simulink model "CORRECTO_REGULADOR"  (R2019b)
settings: Solver=VariableStepAuto  StartTime=0.0  StopTime=50000  RelTol=1e-3
undefined symbols (not defined in the file): n, p1, p2, p3, p6, Vi
libraries: simulink x39
(part 1 of 2)
settings Model: Creator=USUARIO  LastModifiedBy=USUARIO

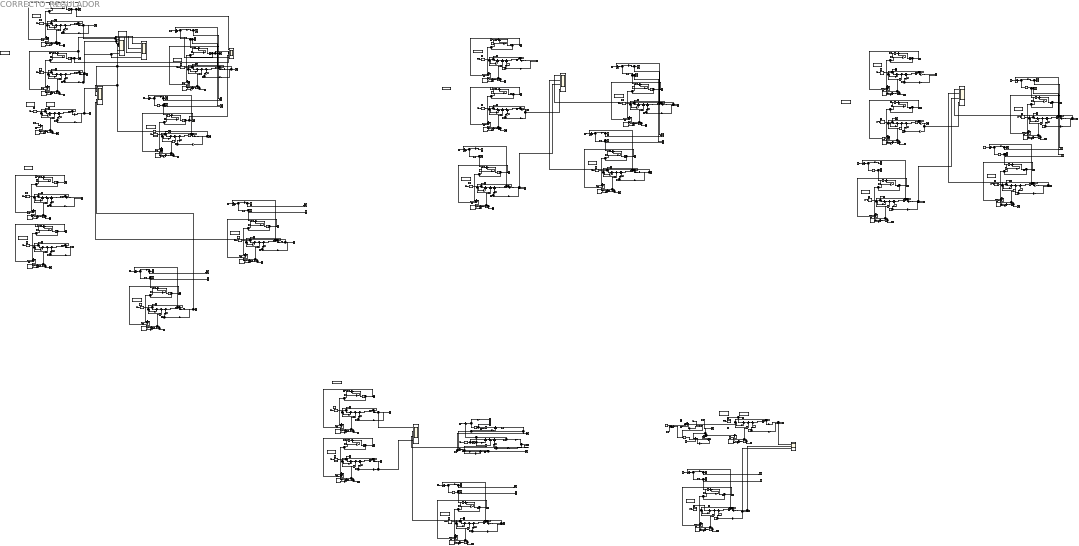
== system CORRECTO_REGULADOR ==
  Clock{,1..25} (26 alike) : Clock
  Constant{1,3,5..7,9,11,15,17,19,21,24,26,28,31,35,37,39,41..43,45..46,48} (24 alike) : Constant  Value=0
  Constant{2,4,8,10,12..14,16,18,20,22..23,25,27,30,32..34,36,38,40,44,47} (23 alike) : Constant  Value=Vi
  Divide{1..23} (23 alike) : Product  Inputs=*/
  Error glucémico{,1,3..4,6,8,12..15,17,19} (12 alike) : Scope
  "Error glucémico   " : Scope
  Error glucémico{2,5,7,9,16,18,20} (7 alike) : Scope  NumInputPorts=2
  Gain{1,6,8,10,15,17,23,26,31,35,37,41,44,52..53,57,63..64,68,73,76,80,83,88,91,95,100,103,105,110,113,118,121,126,129,134,141..142,146,152,155..156,159,164,167,171,173,178,181,185} (50 alike) : Gain  Gain=p1
  Gain{7,16,24,42,45..46,59,74,77..78,81,89,101,104,111,119,127,135,148,153,157,165,172,179,186} (25 alike) : Gain  Gain=p2
  Gain{3,5,9,12,14,18,20,22,25,28,30,33,38,40,43,47,49,51,55,60,62,66,70,72,75,79,82,85,87,90,93,97,99,102,107,109,112,115,117,120,123,125,128,131,133,136,138,140,144,149,151,154,158,161,163,166,169..170,175,177,180,183..184} (63 alike) : Gain  Gain=18
  Gain{2,11,19,27,32,36,48,54,58,65,69,84,92,96,106,114,122,130,137,143,147,160,168,174,182} (25 alike) : Gain  Gain=p3
  Gain{4,13,21,29,34,39,50,56,61,67,71,86,94,98,108,116,124,132,139,145,150,162,176} (23 alike) : Gain  Gain=n
  "Glucosa " : Constant  Value=10
  "Glucosa basal     " : Constant  Value=7
  Glucosa basal{1..14,16..22} (21 alike) : Constant  Value=7
  Glucosa basal23 : Constant  Value=4.5
  Glucosa basal24 : Constant  Value=6
  Glucosa basal25 : Constant  Value=6
  Glucosa basal26 : Constant
  Glucosa basal27 : Constant  Value=0
  Glucosa con regulador : Scope  NumInputPorts=4
  Grafica ingesta D{1..14,16..25} (24 alike) : Scope
  Gráfica de la glucosa : Scope  NumInputPorts=2
  Gráfica de la ingesta : Scope
  Gráfica de la insulina : Scope  NumInputPorts=2
  Gráfica de la insulina activa : Scope
  INSULINA : Scope  NumInputPorts=2
  Ib : Constant  Value=10
  "Ingesta    " : MATLAB Function  TreatAsAtomicUnit=on
  Ingesta 75 g1 : MATLAB Function  TreatAsAtomicUnit=on
  Ingesta 75 g10 : MATLAB Function  TreatAsAtomicUnit=on
  Ingesta 75 g11 : MATLAB Function  TreatAsAtomicUnit=on
  Ingesta 75 g12 : MATLAB Function  TreatAsAtomicUnit=on
  Ingesta 75 g13 : MATLAB Function  TreatAsAtomicUnit=on
  Ingesta 75 g14 : MATLAB Function  TreatAsAtomicUnit=on
  Ingesta 75 g16 : MATLAB Function  TreatAsAtomicUnit=on
  Ingesta 75 g17 : MATLAB Function  TreatAsAtomicUnit=on
  Ingesta 75 g18 : MATLAB Function  TreatAsAtomicUnit=on
  Ingesta 75 g19 : MATLAB Function  TreatAsAtomicUnit=on
  Ingesta 75 g2 : MATLAB Function  TreatAsAtomicUnit=on
  Ingesta 75 g20 : MATLAB Function  TreatAsAtomicUnit=on
  Ingesta 75 g21 : MATLAB Function  TreatAsAtomicUnit=on
  Ingesta 75 g22 : MATLAB Function  TreatAsAtomicUnit=on
  Ingesta 75 g23 : MATLAB Function  TreatAsAtomicUnit=on
  Ingesta 75 g24 : MATLAB Function  TreatAsAtomicUnit=on
  Ingesta 75 g25 : MATLAB Function  TreatAsAtomicUnit=on
  Ingesta 75 g3 : MATLAB Function  TreatAsAtomicUnit=on
  Ingesta 75 g4 : MATLAB Function  TreatAsAtomicUnit=on
  Ingesta 75 g5 : MATLAB Function  TreatAsAtomicUnit=on
  Ingesta 75 g6 : MATLAB Function  TreatAsAtomicUnit=on
  Ingesta 75 g7 : MATLAB Function  TreatAsAtomicUnit=on
  Ingesta 75 g8 : MATLAB Function  TreatAsAtomicUnit=on
  Ingesta 75 g9 : MATLAB Function  TreatAsAtomicUnit=on
  "Insulina basal     " : Constant  Value=10
  Insulina basal{1..14,16..22,24..25} (23 alike) : Constant  Value=10
  Insulina basal23 : Constant  Value=12
  Integrator{1,4,7,9,11,13,16,22,25,28,31,36,39,42..43,46,49,53,56,59,62,64,69} (23 alike) : Integrator  InitialCondition=10
  Integrator{2,5,8,10,14,17,19,23,26,29,32,34,37,40,44,47,50,54,57,60,63,65} (22 alike) : Integrator  InitialCondition=7
  Integrator{3,6,12,18,20..21,27,30,35,41,45,48,51..52,58,61,66,68,71,74} (20 alike) : Integrator
  Integrator{15,24,33,38,55} (5 alike) : Integrator  InitialCondition=-0.000194
  Integrator67 : Integrator  InitialCondition=4.5
  Integrator70 : Integrator  InitialCondition=9.5
  Integrator72 : Integrator  InitialCondition=9.5
  Integrator73 : Integrator  InitialCondition=12
  Model Info1 : simulink/Model-Wide Utilities/Model Info  Frame=on  DisplayStringWithTags=|  HorizontalTextAlignment=Center  LeftAlignmentValue=0.5
      | MODELO MODIFICADO
      | 
      | INGESTA SIN INSULINA
      | 
      | PERSONA DIABETICA tipo 1
  Model Info10 : simulink/Model-Wide Utilities/Model Info  Frame=on  DisplayStringWithTags=|  HorizontalTextAlignment=Center  LeftAlignmentValue=0.5
      | MODELO MODIFICADO
      | 
      | TRAS INGESTA CON INSULINA
      | 
      | PERSONA DIABETICA
  Model Info11 : simulink/Model-Wide Utilities/Model Info  Frame=on  DisplayStringWithTags=|  HorizontalTextAlignment=Center  LeftAlignmentValue=0.5
      | MODELO MODIFICADO
      | 
      | INGESTA SIN INSULINA
      | 
      | PERSONA DIABETICA tipo 1
  Model Info12 : simulink/Model-Wide Utilities/Model Info  Frame=on  DisplayStringWithTags=|  HorizontalTextAlignment=Center  LeftAlignmentValue=0.5
      | MODELO MODIFICADO
      | 
      | INGESTA SIN INSULINA
      | 
      | PERSONA DIABETICA tipo 1
  Model Info13 : simulink/Model-Wide Utilities/Model Info  Frame=on  DisplayStringWithTags=PRUEBA Y ERROR  HorizontalTextAlignment=Center  LeftAlignmentValue=0.5
  Model Info15 : simulink/Model-Wide Utilities/Model Info  Frame=on  DisplayStringWithTags=|  HorizontalTextAlignment=Center  LeftAlignmentValue=0.5
      | MODELO MODIFICADO
      | 
      | INGESTA SIN INSULINA
      | 
      | PERSONA DIABETICA tipo 1
  Model Info16 : simulink/Model-Wide Utilities/Model Info  Frame=on  DisplayStringWithTags=|  HorizontalTextAlignment=Center  LeftAlignmentValue=0.5
      | MODELO MODIFICADO
      | 
      | INGESTA SIN INSULINA
      | 
      | PERSONA DIABETICA tipo 1
  Model Info17 : simulink/Model-Wide Utilities/Model Info  Frame=on  DisplayStringWithTags=|  HorizontalTextAlignment=Center  LeftAlignmentValue=0.5
      | MODELO MODIFICADO
      | 
      | INGESTA SIN INSULINA
      | 
      | PERSONA DIABETICA tipo 1
  Model Info18 : simulink/Model-Wide Utilities/Model Info  Frame=on  DisplayStringWithTags=|  HorizontalTextAlignment=Center  LeftAlignmentValue=0.5
      | MODELO MODIFICADO
      | 
      | INGESTA SIN INSULINA
      | 
      | PERSONA DIABETICA tipo 1
  Model Info19 : simulink/Model-Wide Utilities/Model Info  Frame=on  DisplayStringWithTags=|  HorizontalTextAlignment=Center  LeftAlignmentValue=0.5
      | MODELO MODIFICADO
      | 
      | INGESTA SIN INSULINA
      | 
      | PERSONA DIABETICA tipo 1
  Model Info2 : simulink/Model-Wide Utilities/Model Info  Frame=on  DisplayStringWithTags=|  HorizontalTextAlignment=Center  LeftAlignmentValue=0.5
      | MODELO MODIFICADO
      | 
      | INGESTA SIN INSULINA
      | 
      | PERSONA DIABETICA tipo 1
  Model Info20 : simulink/Model-Wide Utilities/Model Info  Frame=on  DisplayStringWithTags=|  HorizontalTextAlignment=Center  LeftAlignmentValue=0.5
      | MODELO MODIFICADO
      | 
      | INGESTA SIN INSULINA
      | 
      | PERSONA DIABETICA tipo 1
  Model Info21 : simulink/Model-Wide Utilities/Model Info  Frame=on  DisplayStringWithTags=VARIACION TÉRMINO I  HorizontalTextAlignment=Center  LeftAlignmentValue=0.5
  Model Info22 : simulink/Model-Wide Utilities/Model Info  Frame=on  DisplayStringWithTags=|  HorizontalTextAlignment=Center  LeftAlignmentValue=0.5
      | MODELO MODIFICADO
      | 
      | INGESTA SIN INSULINA
      | 
      | PERSONA DIABETICA tipo 1
  Model Info23 : simulink/Model-Wide Utilities/Model Info  Frame=on  DisplayStringWithTags=|  HorizontalTextAlignment=Center  LeftAlignmentValue=0.5
      | Insulina constante 
      | igual a la basal
      | 
      | I(0) = Ib
  Model Info24 : simulink/Model-Wide Utilities/Model Info  Frame=on  DisplayStringWithTags=|  HorizontalTextAlignment=Center  LeftAlignmentValue=0.5
      | MODELO ORIGINAL
      | 
      | 
      | PERSONA NO DIABETICA
      | 
      | CON INSULINA CONSTANTE
  Model Info25 : simulink/Model-Wide Utilities/Model Info  Frame=on  DisplayStringWithTags=|  HorizontalTextAlignment=Center  LeftAlignmentValue=0.5
      | MODELO MODIFICADO
      | 
      | INGESTA SIN INSULINA
      | 
      | PERSONA DIABETICA tipo 1
  Model Info26 : simulink/Model-Wide Utilities/Model Info  Frame=on  DisplayStringWithTags=|  HorizontalTextAlignment=Center  LeftAlignmentValue=0.5
      | Insulina constante 
      | igual a la basal
      | 
      | I(0) = Ib
  Model Info27 : simulink/Model-Wide Utilities/Model Info  Frame=on  DisplayStringWithTags=|  HorizontalTextAlignment=Center  LeftAlignmentValue=0.5
      | MODELO ORIGINAL
      | 
      | 
      | PERSONA NO DIABETICA
      | 
      | CON INSULINA VARIABLE
  Model Info3 : simulink/Model-Wide Utilities/Model Info  Frame=on  DisplayStringWithTags=|  HorizontalTextAlignment=Center  LeftAlignmentValue=0.5
      | MODELO MODIFICADO
      | 
      | INGESTA SIN INSULINA
      | 
      | PERSONA DIABETICA tipo 1
  Model Info4 : simulink/Model-Wide Utilities/Model Info  Frame=on  DisplayStringWithTags=REGULADOR SINTONIZADO  HorizontalTextAlignment=Center  LeftAlignmentValue=0.5
  Model Info5 : simulink/Model-Wide Utilities/Model Info  Frame=on  DisplayStringWithTags=|  HorizontalTextAlignment=Center  LeftAlignmentValue=0.5
      | MODELO MODIFICADO
      | 
      | TRAS INGESTA CON INSULINA
      | 
      | PERSONA DIABETICA
  Model Info6 : simulink/Model-Wide Utilities/Model Info  Frame=on  DisplayStringWithTags=|  HorizontalTextAlignment=Center  LeftAlignmentValue=0.5
      | MODELO MODIFICADO
      | 
      | INGESTA SIN INSULINA
      | 
      | PERSONA DIABETICA tipo 1
  Model Info7 : simulink/Model-Wide Utilities/Model Info  Frame=on  DisplayStringWithTags=|  HorizontalTextAlignment=Center  LeftAlignmentValue=0.5
      | MODELO MODIFICADO
      | 
      | INGESTA SIN INSULINA
      | 
      | PERSONA DIABETICA tipo 1
  Model Info8 : simulink/Model-Wide Utilities/Model Info  Frame=on  DisplayStringWithTags=VARAICION TERMINO P  HorizontalTextAlignment=Center  LeftAlignmentValue=0.5
  Model Info9 : simulink/Model-Wide Utilities/Model Info  Frame=on  DisplayStringWithTags=REGULADOR SINTONIZADO  HorizontalTextAlignment=Center  LeftAlignmentValue=0.5
  PID Controller : simulink/Continuous/PID Controller  Controller=PID  Form=Ideal  TimeDomain=Continuous-time  SampleTime=-1  IntegratorMethod=Forward Euler  FilterMethod=Forward Euler  ControllerParametersSource=internal  P=-0.4  I=0  D=0  UseFilter=on  N=10  TunerSelectOption=Transfer Function Based (PID Tuner App)  InitialConditionSource=internal  InitialConditionForIntegrator=-0.1  InitialConditionForFilter=0  DifferentiatorICPrevScaledInput=0  ExternalReset=none  TrackingMode=off  Kt=1  LimitOutput=off  UpperSaturationLimit=inf  LowerSaturationLimit=-inf  LinearizeAsGain=on  AntiWindupMode=none  Kb=1  POutMin=[]  POutMax=[]  IOutMin=[]  IOutMax=[]  DOutMin=[]  DOutMax=[]  NOutMin=[]  NOutMax=[]  SumOutMin=[]  SumOutMax=[]  SaturationOutMin=[]  SaturationOutMax=[]  PParamMin=[]  PParamMax=[]  IParamMin=[]  IParamMax=[]  DParamMin=[]  DParamMax=[]  NParamMin=[]  NParamMax=[]  KbParamMin=[]  KbParamMax=[]  KtParamMin=[]  KtParamMax=[]  KbOutMin=[]  KbOutMax=[]  KtOutMin=[]  KtOutMax=[]  IntegratorOutMin=[]  IntegratorOutMax=[]  FilterOutMin=[]  FilterOutMax=[]  SumI1OutMin=[]  SumI1OutMax=[]  SumI2OutMin=[]  SumI2OutMax=[]  SumI3OutMin=[]  SumI3OutMax=[]  SumI4OutMin=[]  SumI4OutMax=[]  SumDOutMin=[]  SumDOutMax=[]  DifferentiatorOutMin=[]  DifferentiatorOutMax=[]  FilterDiffOutCoefMin=[]  FilterDiffOutCoefMax=[]  ReciprocalOutMin=[]  ReciprocalOutMax=[]  SumDenOutMin=[]  SumDenOutMax=[]  SumNumOutMin=[]  SumNumOutMax=[]  DivideOutMin=[]  DivideOutMax=[]  IntegratorContinuousStateAttributes=''  IntegratorStateMustResolveToSignalObject=off  IntegratorRTWStateStorageClass=Auto  FilterContinuousStateAttributes=''  FilterStateMustResolveToSignalObject=off  FilterRTWStateStorageClass=Auto  ParallelPVariant=Passthrough  IdealPVariant=InternalParameters  IVariant=InternalParameters  DVariant=InternalParameters  IntegratorVariant=Continuous  SatVariant=Disabled  AWVariant=Passthrough  PCopyVariant=Disabled  TRVariant=Disabled  FdbkBlocksVariant=Forward  IdealPFdbkVariant=Disabled  SatFdbkVariant=Disabled  DerivativeFilterVariant=ContFilter  NVariant=InternalParameters  NCopyVariant=Disabled  FilterICVariant=InternalICsFilter  IntegratorICVariant=InternalICs  ExternalResetVariant=Disabled  TRSumVariant=Passthrough  SumFdbkVariant=Disabled  SumVariant=Sum_PID
  PID Controller1 : simulink/Continuous/PID Controller  Controller=PID  Form=Ideal  TimeDomain=Continuous-time  SampleTime=-1  IntegratorMethod=Forward Euler  FilterMethod=Forward Euler  ControllerParametersSource=internal  P=-0.4  I=0.00006  D=0  UseFilter=on  N=100  TunerSelectOption=Transfer Function Based (PID Tuner App)  InitialConditionSource=internal  InitialConditionForIntegrator=-0.1  InitialConditionForFilter=0  DifferentiatorICPrevScaledInput=0  ExternalReset=none  TrackingMode=off  Kt=1  LimitOutput=off  UpperSaturationLimit=inf  LowerSaturationLimit=-inf  LinearizeAsGain=on  AntiWindupMode=none  Kb=1  POutMin=[]  POutMax=[]  IOutMin=[]  IOutMax=[]  DOutMin=[]  DOutMax=[]  NOutMin=[]  NOutMax=[]  SumOutMin=[]  SumOutMax=[]  SaturationOutMin=[]  SaturationOutMax=[]  PParamMin=[]  PParamMax=[]  IParamMin=[]  IParamMax=[]  DParamMin=[]  DParamMax=[]  NParamMin=[]  NParamMax=[]  KbParamMin=[]  KbParamMax=[]  KtParamMin=[]  KtParamMax=[]  KbOutMin=[]  KbOutMax=[]  KtOutMin=[]  KtOutMax=[]  IntegratorOutMin=[]  IntegratorOutMax=[]  FilterOutMin=[]  FilterOutMax=[]  SumI1OutMin=[]  SumI1OutMax=[]  SumI2OutMin=[]  SumI2OutMax=[]  SumI3OutMin=[]  SumI3OutMax=[]  SumI4OutMin=[]  SumI4OutMax=[]  SumDOutMin=[]  SumDOutMax=[]  DifferentiatorOutMin=[]  DifferentiatorOutMax=[]  FilterDiffOutCoefMin=[]  FilterDiffOutCoefMax=[]  ReciprocalOutMin=[]  ReciprocalOutMax=[]  SumDenOutMin=[]  SumDenOutMax=[]  SumNumOutMin=[]  SumNumOutMax=[]  DivideOutMin=[]  DivideOutMax=[]  IntegratorContinuousStateAttributes=''  IntegratorStateMustResolveToSignalObject=off  IntegratorRTWStateStorageClass=Auto  FilterContinuousStateAttributes=''  FilterStateMustResolveToSignalObject=off  FilterRTWStateStorageClass=Auto  ParallelPVariant=Passthrough  IdealPVariant=InternalParameters  IVariant=InternalParameters  DVariant=InternalParameters  IntegratorVariant=Continuous  SatVariant=Disabled  AWVariant=Passthrough  PCopyVariant=Disabled  TRVariant=Disabled  FdbkBlocksVariant=Forward  IdealPFdbkVariant=Disabled  SatFdbkVariant=Disabled  DerivativeFilterVariant=ContFilter  NVariant=InternalParameters  NCopyVariant=Disabled  FilterICVariant=InternalICsFilter  IntegratorICVariant=InternalICs  ExternalResetVariant=Disabled  TRSumVariant=Passthrough  SumFdbkVariant=Disabled  SumVariant=Sum_PID
  PID Controller10 : simulink/Continuous/PID Controller  Controller=PID  Form=Ideal  TimeDomain=Continuous-time  SampleTime=-1  IntegratorMethod=Forward Euler  FilterMethod=Forward Euler  ControllerParametersSource=internal  P=-0.4  I=0.00001  D=0  UseFilter=on  N=100  TunerSelectOption=Transfer Function Based (PID Tuner App)  InitialConditionSource=internal  InitialConditionForIntegrator=-0.1  InitialConditionForFilter=0  DifferentiatorICPrevScaledInput=0  ExternalReset=none  TrackingMode=off  Kt=1  LimitOutput=off  UpperSaturationLimit=inf  LowerSaturationLimit=-inf  LinearizeAsGain=on  AntiWindupMode=none  Kb=1  POutMin=[]  POutMax=[]  IOutMin=[]  IOutMax=[]  DOutMin=[]  DOutMax=[]  NOutMin=[]  NOutMax=[]  SumOutMin=[]  SumOutMax=[]  SaturationOutMin=[]  SaturationOutMax=[]  PParamMin=[]  PParamMax=[]  IParamMin=[]  IParamMax=[]  DParamMin=[]  DParamMax=[]  NParamMin=[]  NParamMax=[]  KbParamMin=[]  KbParamMax=[]  KtParamMin=[]  KtParamMax=[]  KbOutMin=[]  KbOutMax=[]  KtOutMin=[]  KtOutMax=[]  IntegratorOutMin=[]  IntegratorOutMax=[]  FilterOutMin=[]  FilterOutMax=[]  SumI1OutMin=[]  SumI1OutMax=[]  SumI2OutMin=[]  SumI2OutMax=[]  SumI3OutMin=[]  SumI3OutMax=[]  SumI4OutMin=[]  SumI4OutMax=[]  SumDOutMin=[]  SumDOutMax=[]  DifferentiatorOutMin=[]  DifferentiatorOutMax=[]  FilterDiffOutCoefMin=[]  FilterDiffOutCoefMax=[]  ReciprocalOutMin=[]  ReciprocalOutMax=[]  SumDenOutMin=[]  SumDenOutMax=[]  SumNumOutMin=[]  SumNumOutMax=[]  DivideOutMin=[]  DivideOutMax=[]  IntegratorContinuousStateAttributes=''  IntegratorStateMustResolveToSignalObject=off  IntegratorRTWStateStorageClass=Auto  FilterContinuousStateAttributes=''  FilterStateMustResolveToSignalObject=off  FilterRTWStateStorageClass=Auto  ParallelPVariant=Passthrough  IdealPVariant=InternalParameters  IVariant=InternalParameters  DVariant=InternalParameters  IntegratorVariant=Continuous  SatVariant=Disabled  AWVariant=Passthrough  PCopyVariant=Disabled  TRVariant=Disabled  FdbkBlocksVariant=Forward  IdealPFdbkVariant=Disabled  SatFdbkVariant=Disabled  DerivativeFilterVariant=ContFilter  NVariant=InternalParameters  NCopyVariant=Disabled  FilterICVariant=InternalICsFilter  IntegratorICVariant=InternalICs  ExternalResetVariant=Disabled  TRSumVariant=Passthrough  SumFdbkVariant=Disabled  SumVariant=Sum_PID
  PID Controller11 : simulink/Continuous/PID Controller  Controller=PID  Form=Ideal  TimeDomain=Continuous-time  SampleTime=-1  IntegratorMethod=Forward Euler  FilterMethod=Forward Euler  ControllerParametersSource=internal  P=-0.49  I=0.0000436  D=477  UseFilter=on  N=100  TunerSelectOption=Transfer Function Based (PID Tuner App)  InitialConditionSource=internal  InitialConditionForIntegrator=-0.1  InitialConditionForFilter=0  DifferentiatorICPrevScaledInput=0  ExternalReset=none  TrackingMode=off  Kt=1  LimitOutput=off  UpperSaturationLimit=inf  LowerSaturationLimit=-inf  LinearizeAsGain=on  AntiWindupMode=none  Kb=1  POutMin=[]  POutMax=[]  IOutMin=[]  IOutMax=[]  DOutMin=[]  DOutMax=[]  NOutMin=[]  NOutMax=[]  SumOutMin=[]  SumOutMax=[]  SaturationOutMin=[]  SaturationOutMax=[]  PParamMin=[]  PParamMax=[]  IParamMin=[]  IParamMax=[]  DParamMin=[]  DParamMax=[]  NParamMin=[]  NParamMax=[]  KbParamMin=[]  KbParamMax=[]  KtParamMin=[]  KtParamMax=[]  KbOutMin=[]  KbOutMax=[]  KtOutMin=[]  KtOutMax=[]  IntegratorOutMin=[]  IntegratorOutMax=[]  FilterOutMin=[]  FilterOutMax=[]  SumI1OutMin=[]  SumI1OutMax=[]  SumI2OutMin=[]  SumI2OutMax=[]  SumI3OutMin=[]  SumI3OutMax=[]  SumI4OutMin=[]  SumI4OutMax=[]  SumDOutMin=[]  SumDOutMax=[]  DifferentiatorOutMin=[]  DifferentiatorOutMax=[]  FilterDiffOutCoefMin=[]  FilterDiffOutCoefMax=[]  ReciprocalOutMin=[]  ReciprocalOutMax=[]  SumDenOutMin=[]  SumDenOutMax=[]  SumNumOutMin=[]  SumNumOutMax=[]  DivideOutMin=[]  DivideOutMax=[]  IntegratorContinuousStateAttributes=''  IntegratorStateMustResolveToSignalObject=off  IntegratorRTWStateStorageClass=Auto  FilterContinuousStateAttributes=''  FilterStateMustResolveToSignalObject=off  FilterRTWStateStorageClass=Auto  ParallelPVariant=Passthrough  IdealPVariant=InternalParameters  IVariant=InternalParameters  DVariant=InternalParameters  IntegratorVariant=Continuous  SatVariant=Disabled  AWVariant=Passthrough  PCopyVariant=Disabled  TRVariant=Disabled  FdbkBlocksVariant=Forward  IdealPFdbkVariant=Disabled  SatFdbkVariant=Disabled  DerivativeFilterVariant=ContFilter  NVariant=InternalParameters  NCopyVariant=Disabled  FilterICVariant=InternalICsFilter  IntegratorICVariant=InternalICs  ExternalResetVariant=Disabled  TRSumVariant=Passthrough  SumFdbkVariant=Disabled  SumVariant=Sum_PID
  PID Controller12 : simulink/Continuous/PID Controller  Controller=PID  Form=Ideal  TimeDomain=Continuous-time  SampleTime=-1  IntegratorMethod=Forward Euler  FilterMethod=Forward Euler  ControllerParametersSource=internal  P=-0.49  I=0.00004  D=477  UseFilter=on  N=100  TunerSelectOption=Transfer Function Based (PID Tuner App)  InitialConditionSource=internal  InitialConditionForIntegrator=-0.1  InitialConditionForFilter=0  DifferentiatorICPrevScaledInput=0  ExternalReset=none  TrackingMode=off  Kt=1  LimitOutput=off  UpperSaturationLimit=inf  LowerSaturationLimit=-inf  LinearizeAsGain=on  AntiWindupMode=none  Kb=1  POutMin=[]  POutMax=[]  IOutMin=[]  IOutMax=[]  DOutMin=[]  DOutMax=[]  NOutMin=[]  NOutMax=[]  SumOutMin=[]  SumOutMax=[]  SaturationOutMin=[]  SaturationOutMax=[]  PParamMin=[]  PParamMax=[]  IParamMin=[]  IParamMax=[]  DParamMin=[]  DParamMax=[]  NParamMin=[]  NParamMax=[]  KbParamMin=[]  KbParamMax=[]  KtParamMin=[]  KtParamMax=[]  KbOutMin=[]  KbOutMax=[]  KtOutMin=[]  KtOutMax=[]  IntegratorOutMin=[]  IntegratorOutMax=[]  FilterOutMin=[]  FilterOutMax=[]  SumI1OutMin=[]  SumI1OutMax=[]  SumI2OutMin=[]  SumI2OutMax=[]  SumI3OutMin=[]  SumI3OutMax=[]  SumI4OutMin=[]  SumI4OutMax=[]  SumDOutMin=[]  SumDOutMax=[]  DifferentiatorOutMin=[]  DifferentiatorOutMax=[]  FilterDiffOutCoefMin=[]  FilterDiffOutCoefMax=[]  ReciprocalOutMin=[]  ReciprocalOutMax=[]  SumDenOutMin=[]  SumDenOutMax=[]  SumNumOutMin=[]  SumNumOutMax=[]  DivideOutMin=[]  DivideOutMax=[]  IntegratorContinuousStateAttributes=''  IntegratorStateMustResolveToSignalObject=off  IntegratorRTWStateStorageClass=Auto  FilterContinuousStateAttributes=''  FilterStateMustResolveToSignalObject=off  FilterRTWStateStorageClass=Auto  ParallelPVariant=Passthrough  IdealPVariant=InternalParameters  IVariant=InternalParameters  DVariant=InternalParameters  IntegratorVariant=Continuous  SatVariant=Disabled  AWVariant=Passthrough  PCopyVariant=Disabled  TRVariant=Disabled  FdbkBlocksVariant=Forward  IdealPFdbkVariant=Disabled  SatFdbkVariant=Disabled  DerivativeFilterVariant=ContFilter  NVariant=InternalParameters  NCopyVariant=Disabled  FilterICVariant=InternalICsFilter  IntegratorICVariant=InternalICs  ExternalResetVariant=Disabled  TRSumVariant=Passthrough  SumFdbkVariant=Disabled  SumVariant=Sum_PID
  PID Controller2 : simulink/Continuous/PID Controller  Controller=PID  Form=Ideal  TimeDomain=Continuous-time  SampleTime=-1  IntegratorMethod=Forward Euler  FilterMethod=Forward Euler  ControllerParametersSource=internal  P=-0.4  I=0.00003  D=0  UseFilter=on  N=10  TunerSelectOption=Transfer Function Based (PID Tuner App)  InitialConditionSource=internal  InitialConditionForIntegrator=-0.1  InitialConditionForFilter=0  DifferentiatorICPrevScaledInput=0  ExternalReset=none  TrackingMode=off  Kt=1  LimitOutput=off  UpperSaturationLimit=inf  LowerSaturationLimit=-inf  LinearizeAsGain=on  AntiWindupMode=none  Kb=1  POutMin=[]  POutMax=[]  IOutMin=[]  IOutMax=[]  DOutMin=[]  DOutMax=[]  NOutMin=[]  NOutMax=[]  SumOutMin=[]  SumOutMax=[]  SaturationOutMin=[]  SaturationOutMax=[]  PParamMin=[]  PParamMax=[]  IParamMin=[]  IParamMax=[]  DParamMin=[]  DParamMax=[]  NParamMin=[]  NParamMax=[]  KbParamMin=[]  KbParamMax=[]  KtParamMin=[]  KtParamMax=[]  KbOutMin=[]  KbOutMax=[]  KtOutMin=[]  KtOutMax=[]  IntegratorOutMin=[]  IntegratorOutMax=[]  FilterOutMin=[]  FilterOutMax=[]  SumI1OutMin=[]  SumI1OutMax=[]  SumI2OutMin=[]  SumI2OutMax=[]  SumI3OutMin=[]  SumI3OutMax=[]  SumI4OutMin=[]  SumI4OutMax=[]  SumDOutMin=[]  SumDOutMax=[]  DifferentiatorOutMin=[]  DifferentiatorOutMax=[]  FilterDiffOutCoefMin=[]  FilterDiffOutCoefMax=[]  ReciprocalOutMin=[]  ReciprocalOutMax=[]  SumDenOutMin=[]  SumDenOutMax=[]  SumNumOutMin=[]  SumNumOutMax=[]  DivideOutMin=[]  DivideOutMax=[]  IntegratorContinuousStateAttributes=''  IntegratorStateMustResolveToSignalObject=off  IntegratorRTWStateStorageClass=Auto  FilterContinuousStateAttributes=''  FilterStateMustResolveToSignalObject=off  FilterRTWStateStorageClass=Auto  ParallelPVariant=Passthrough  IdealPVariant=InternalParameters  IVariant=InternalParameters  DVariant=InternalParameters  IntegratorVariant=Continuous  SatVariant=Disabled  AWVariant=Passthrough  PCopyVariant=Disabled  TRVariant=Disabled  FdbkBlocksVariant=Forward  IdealPFdbkVariant=Disabled  SatFdbkVariant=Disabled  DerivativeFilterVariant=ContFilter  NVariant=InternalParameters  NCopyVariant=Disabled  FilterICVariant=InternalICsFilter  IntegratorICVariant=InternalICs  ExternalResetVariant=Disabled  TRSumVariant=Passthrough  SumFdbkVariant=Disabled  SumVariant=Sum_PID
  PID Controller3 : simulink/Continuous/PID Controller  Controller=PID  Form=Ideal  TimeDomain=Continuous-time  SampleTime=-1  IntegratorMethod=Forward Euler  FilterMethod=Forward Euler  ControllerParametersSource=internal  P=-0.3195  I=0.000033  D=0  UseFilter=on  N=100  TunerSelectOption=Transfer Function Based (PID Tuner App)  InitialConditionSource=internal  InitialConditionForIntegrator=-0.1  InitialConditionForFilter=0  DifferentiatorICPrevScaledInput=0  ExternalReset=none  TrackingMode=off  Kt=1  LimitOutput=off  UpperSaturationLimit=inf  LowerSaturationLimit=-inf  LinearizeAsGain=on  AntiWindupMode=none  Kb=1  POutMin=[]  POutMax=[]  IOutMin=[]  IOutMax=[]  DOutMin=[]  DOutMax=[]  NOutMin=[]  NOutMax=[]  SumOutMin=[]  SumOutMax=[]  SaturationOutMin=[]  SaturationOutMax=[]  PParamMin=[]  PParamMax=[]  IParamMin=[]  IParamMax=[]  DParamMin=[]  DParamMax=[]  NParamMin=[]  NParamMax=[]  KbParamMin=[]  KbParamMax=[]  KtParamMin=[]  KtParamMax=[]  KbOutMin=[]  KbOutMax=[]  KtOutMin=[]  KtOutMax=[]  IntegratorOutMin=[]  IntegratorOutMax=[]  FilterOutMin=[]  FilterOutMax=[]  SumI1OutMin=[]  SumI1OutMax=[]  SumI2OutMin=[]  SumI2OutMax=[]  SumI3OutMin=[]  SumI3OutMax=[]  SumI4OutMin=[]  SumI4OutMax=[]  SumDOutMin=[]  SumDOutMax=[]  DifferentiatorOutMin=[]  DifferentiatorOutMax=[]  FilterDiffOutCoefMin=[]  FilterDiffOutCoefMax=[]  ReciprocalOutMin=[]  ReciprocalOutMax=[]  SumDenOutMin=[]  SumDenOutMax=[]  SumNumOutMin=[]  SumNumOutMax=[]  DivideOutMin=[]  DivideOutMax=[]  IntegratorContinuousStateAttributes=''  IntegratorStateMustResolveToSignalObject=off  IntegratorRTWStateStorageClass=Auto  FilterContinuousStateAttributes=''  FilterStateMustResolveToSignalObject=off  FilterRTWStateStorageClass=Auto  ParallelPVariant=Passthrough  IdealPVariant=InternalParameters  IVariant=InternalParameters  DVariant=InternalParameters  IntegratorVariant=Continuous  SatVariant=Disabled  AWVariant=Passthrough  PCopyVariant=Disabled  TRVariant=Disabled  FdbkBlocksVariant=Forward  IdealPFdbkVariant=Disabled  SatFdbkVariant=Disabled  DerivativeFilterVariant=ContFilter  NVariant=InternalParameters  NCopyVariant=Disabled  FilterICVariant=InternalICsFilter  IntegratorICVariant=InternalICs  ExternalResetVariant=Disabled  TRSumVariant=Passthrough  SumFdbkVariant=Disabled  SumVariant=Sum_PID
  PID Controller4 : simulink/Continuous/PID Controller  Controller=PID  Form=Ideal  TimeDomain=Continuous-time  SampleTime=-1  IntegratorMethod=Forward Euler  FilterMethod=Forward Euler  ControllerParametersSource=internal  P=-0.1  I=0.00003  D=0  UseFilter=on  N=100  TunerSelectOption=Transfer Function Based (PID Tuner App)  InitialConditionSource=internal  InitialConditionForIntegrator=-0.1  InitialConditionForFilter=0  DifferentiatorICPrevScaledInput=0  ExternalReset=none  TrackingMode=off  Kt=1  LimitOutput=off  UpperSaturationLimit=inf  LowerSaturationLimit=-inf  LinearizeAsGain=on  AntiWindupMode=none  Kb=1  POutMin=[]  POutMax=[]  IOutMin=[]  IOutMax=[]  DOutMin=[]  DOutMax=[]  NOutMin=[]  NOutMax=[]  SumOutMin=[]  SumOutMax=[]  SaturationOutMin=[]  SaturationOutMax=[]  PParamMin=[]  PParamMax=[]  IParamMin=[]  IParamMax=[]  DParamMin=[]  DParamMax=[]  NParamMin=[]  NParamMax=[]  KbParamMin=[]  KbParamMax=[]  KtParamMin=[]  KtParamMax=[]  KbOutMin=[]  KbOutMax=[]  KtOutMin=[]  KtOutMax=[]  IntegratorOutMin=[]  IntegratorOutMax=[]  FilterOutMin=[]  FilterOutMax=[]  SumI1OutMin=[]  SumI1OutMax=[]  SumI2OutMin=[]  SumI2OutMax=[]  SumI3OutMin=[]  SumI3OutMax=[]  SumI4OutMin=[]  SumI4OutMax=[]  SumDOutMin=[]  SumDOutMax=[]  DifferentiatorOutMin=[]  DifferentiatorOutMax=[]  FilterDiffOutCoefMin=[]  FilterDiffOutCoefMax=[]  ReciprocalOutMin=[]  ReciprocalOutMax=[]  SumDenOutMin=[]  SumDenOutMax=[]  SumNumOutMin=[]  SumNumOutMax=[]  DivideOutMin=[]  DivideOutMax=[]  IntegratorContinuousStateAttributes=''  IntegratorStateMustResolveToSignalObject=off  IntegratorRTWStateStorageClass=Auto  FilterContinuousStateAttributes=''  FilterStateMustResolveToSignalObject=off  FilterRTWStateStorageClass=Auto  ParallelPVariant=Passthrough  IdealPVariant=InternalParameters  IVariant=InternalParameters  DVariant=InternalParameters  IntegratorVariant=Continuous  SatVariant=Disabled  AWVariant=Passthrough  PCopyVariant=Disabled  TRVariant=Disabled  FdbkBlocksVariant=Forward  IdealPFdbkVariant=Disabled  SatFdbkVariant=Disabled  DerivativeFilterVariant=ContFilter  NVariant=InternalParameters  NCopyVariant=Disabled  FilterICVariant=InternalICsFilter  IntegratorICVariant=InternalICs  ExternalResetVariant=Disabled  TRSumVariant=Passthrough  SumFdbkVariant=Disabled  SumVariant=Sum_PID
  PID Controller5 : simulink/Continuous/PID Controller  Controller=PID  Form=Ideal  TimeDomain=Continuous-time  SampleTime=-1  IntegratorMethod=Forward Euler  FilterMethod=Forward Euler  ControllerParametersSource=internal  P=-0.3195  I=0.000033  D=0  UseFilter=on  N=100  TunerSelectOption=Transfer Function Based (PID Tuner App)  InitialConditionSource=internal  InitialConditionForIntegrator=-0.1  InitialConditionForFilter=0  DifferentiatorICPrevScaledInput=0  ExternalReset=none  TrackingMode=off  Kt=1  LimitOutput=off  UpperSaturationLimit=inf  LowerSaturationLimit=-inf  LinearizeAsGain=on  AntiWindupMode=none  Kb=1  POutMin=[]  POutMax=[]  IOutMin=[]  IOutMax=[]  DOutMin=[]  DOutMax=[]  NOutMin=[]  NOutMax=[]  SumOutMin=[]  SumOutMax=[]  SaturationOutMin=[]  SaturationOutMax=[]  PParamMin=[]  PParamMax=[]  IParamMin=[]  IParamMax=[]  DParamMin=[]  DParamMax=[]  NParamMin=[]  NParamMax=[]  KbParamMin=[]  KbParamMax=[]  KtParamMin=[]  KtParamMax=[]  KbOutMin=[]  KbOutMax=[]  KtOutMin=[]  KtOutMax=[]  IntegratorOutMin=[]  IntegratorOutMax=[]  FilterOutMin=[]  FilterOutMax=[]  SumI1OutMin=[]  SumI1OutMax=[]  SumI2OutMin=[]  SumI2OutMax=[]  SumI3OutMin=[]  SumI3OutMax=[]  SumI4OutMin=[]  SumI4OutMax=[]  SumDOutMin=[]  SumDOutMax=[]  DifferentiatorOutMin=[]  DifferentiatorOutMax=[]  FilterDiffOutCoefMin=[]  FilterDiffOutCoefMax=[]  ReciprocalOutMin=[]  ReciprocalOutMax=[]  SumDenOutMin=[]  SumDenOutMax=[]  SumNumOutMin=[]  SumNumOutMax=[]  DivideOutMin=[]  DivideOutMax=[]  IntegratorContinuousStateAttributes=''  IntegratorStateMustResolveToSignalObject=off  IntegratorRTWStateStorageClass=Auto  FilterContinuousStateAttributes=''  FilterStateMustResolveToSignalObject=off  FilterRTWStateStorageClass=Auto  ParallelPVariant=Passthrough  IdealPVariant=InternalParameters  IVariant=InternalParameters  DVariant=InternalParameters  IntegratorVariant=Continuous  SatVariant=Disabled  AWVariant=Passthrough  PCopyVariant=Disabled  TRVariant=Disabled  FdbkBlocksVariant=Forward  IdealPFdbkVariant=Disabled  SatFdbkVariant=Disabled  DerivativeFilterVariant=ContFilter  NVariant=InternalParameters  NCopyVariant=Disabled  FilterICVariant=InternalICsFilter  IntegratorICVariant=InternalICs  ExternalResetVariant=Disabled  TRSumVariant=Passthrough  SumFdbkVariant=Disabled  SumVariant=Sum_PID
  PID Controller6 : simulink/Continuous/PID Controller  Controller=PID  Form=Ideal  TimeDomain=Continuous-time  SampleTime=-1  IntegratorMethod=Forward Euler  FilterMethod=Forward Euler  ControllerParametersSource=internal  P=-0.49  I=0.00004  D=477  UseFilter=on  N=100  TunerSelectOption=Transfer Function Based (PID Tuner App)  InitialConditionSource=internal  InitialConditionForIntegrator=-0.1  InitialConditionForFilter=0  DifferentiatorICPrevScaledInput=0  ExternalReset=none  TrackingMode=off  Kt=1  LimitOutput=off  UpperSaturationLimit=inf  LowerSaturationLimit=-inf  LinearizeAsGain=on  AntiWindupMode=none  Kb=1  POutMin=[]  POutMax=[]  IOutMin=[]  IOutMax=[]  DOutMin=[]  DOutMax=[]  NOutMin=[]  NOutMax=[]  SumOutMin=[]  SumOutMax=[]  SaturationOutMin=[]  SaturationOutMax=[]  PParamMin=[]  PParamMax=[]  IParamMin=[]  IParamMax=[]  DParamMin=[]  DParamMax=[]  NParamMin=[]  NParamMax=[]  KbParamMin=[]  KbParamMax=[]  KtParamMin=[]  KtParamMax=[]  KbOutMin=[]  KbOutMax=[]  KtOutMin=[]  KtOutMax=[]  IntegratorOutMin=[]  IntegratorOutMax=[]  FilterOutMin=[]  FilterOutMax=[]  SumI1OutMin=[]  SumI1OutMax=[]  SumI2OutMin=[]  SumI2OutMax=[]  SumI3OutMin=[]  SumI3OutMax=[]  SumI4OutMin=[]  SumI4OutMax=[]  SumDOutMin=[]  SumDOutMax=[]  DifferentiatorOutMin=[]  DifferentiatorOutMax=[]  FilterDiffOutCoefMin=[]  FilterDiffOutCoefMax=[]  ReciprocalOutMin=[]  ReciprocalOutMax=[]  SumDenOutMin=[]  SumDenOutMax=[]  SumNumOutMin=[]  SumNumOutMax=[]  DivideOutMin=[]  DivideOutMax=[]  IntegratorContinuousStateAttributes=''  IntegratorStateMustResolveToSignalObject=off  IntegratorRTWStateStorageClass=Auto  FilterContinuousStateAttributes=''  FilterStateMustResolveToSignalObject=off  FilterRTWStateStorageClass=Auto  ParallelPVariant=Passthrough  IdealPVariant=InternalParameters  IVariant=InternalParameters  DVariant=InternalParameters  IntegratorVariant=Continuous  SatVariant=Disabled  AWVariant=Passthrough  PCopyVariant=Disabled  TRVariant=Disabled  FdbkBlocksVariant=Forward  IdealPFdbkVariant=Disabled  SatFdbkVariant=Disabled  DerivativeFilterVariant=ContFilter  NVariant=InternalParameters  NCopyVariant=Disabled  FilterICVariant=InternalICsFilter  IntegratorICVariant=InternalICs  ExternalResetVariant=Disabled  TRSumVariant=Passthrough  SumFdbkVariant=Disabled  SumVariant=Sum_PID
  PID Controller7 : simulink/Continuous/PID Controller  Controller=PID  Form=Ideal  TimeDomain=Continuous-time  SampleTime=-1  IntegratorMethod=Forward Euler  FilterMethod=Forward Euler  ControllerParametersSource=internal  P=-0.7  I=0.00003  D=0  UseFilter=on  N=100  TunerSelectOption=Transfer Function Based (PID Tuner App)  InitialConditionSource=internal  InitialConditionForIntegrator=-0.1  InitialConditionForFilter=0  DifferentiatorICPrevScaledInput=0  ExternalReset=none  TrackingMode=off  Kt=1  LimitOutput=off  UpperSaturationLimit=inf  LowerSaturationLimit=-inf  LinearizeAsGain=on  AntiWindupMode=none  Kb=1  POutMin=[]  POutMax=[]  IOutMin=[]  IOutMax=[]  DOutMin=[]  DOutMax=[]  NOutMin=[]  NOutMax=[]  SumOutMin=[]  SumOutMax=[]  SaturationOutMin=[]  SaturationOutMax=[]  PParamMin=[]  PParamMax=[]  IParamMin=[]  IParamMax=[]  DParamMin=[]  DParamMax=[]  NParamMin=[]  NParamMax=[]  KbParamMin=[]  KbParamMax=[]  KtParamMin=[]  KtParamMax=[]  KbOutMin=[]  KbOutMax=[]  KtOutMin=[]  KtOutMax=[]  IntegratorOutMin=[]  IntegratorOutMax=[]  FilterOutMin=[]  FilterOutMax=[]  SumI1OutMin=[]  SumI1OutMax=[]  SumI2OutMin=[]  SumI2OutMax=[]  SumI3OutMin=[]  SumI3OutMax=[]  SumI4OutMin=[]  SumI4OutMax=[]  SumDOutMin=[]  SumDOutMax=[]  DifferentiatorOutMin=[]  DifferentiatorOutMax=[]  FilterDiffOutCoefMin=[]  FilterDiffOutCoefMax=[]  ReciprocalOutMin=[]  ReciprocalOutMax=[]  SumDenOutMin=[]  SumDenOutMax=[]  SumNumOutMin=[]  SumNumOutMax=[]  DivideOutMin=[]  DivideOutMax=[]  IntegratorContinuousStateAttributes=''  IntegratorStateMustResolveToSignalObject=off  IntegratorRTWStateStorageClass=Auto  FilterContinuousStateAttributes=''  FilterStateMustResolveToSignalObject=off  FilterRTWStateStorageClass=Auto  ParallelPVariant=Passthrough  IdealPVariant=InternalParameters  IVariant=InternalParameters  DVariant=InternalParameters  IntegratorVariant=Continuous  SatVariant=Disabled  AWVariant=Passthrough  PCopyVariant=Disabled  TRVariant=Disabled  FdbkBlocksVariant=Forward  IdealPFdbkVariant=Disabled  SatFdbkVariant=Disabled  DerivativeFilterVariant=ContFilter  NVariant=InternalParameters  NCopyVariant=Disabled  FilterICVariant=InternalICsFilter  IntegratorICVariant=InternalICs  ExternalResetVariant=Disabled  TRSumVariant=Passthrough  SumFdbkVariant=Disabled  SumVariant=Sum_PID
  PID Controller8 : simulink/Continuous/PID Controller  Controller=PID  Form=Ideal  TimeDomain=Continuous-time  SampleTime=-1  IntegratorMethod=Forward Euler  FilterMethod=Forward Euler  ControllerParametersSource=internal  P=-0.4  I=0.00006  D=0  UseFilter=on  N=10  TunerSelectOption=Transfer Function Based (PID Tuner App)  InitialConditionSource=internal  InitialConditionForIntegrator=-0.1  InitialConditionForFilter=0  DifferentiatorICPrevScaledInput=0  ExternalReset=none  TrackingMode=off  Kt=1  LimitOutput=off  UpperSaturationLimit=inf  LowerSaturationLimit=-inf  LinearizeAsGain=on  AntiWindupMode=none  Kb=1  POutMin=[]  POutMax=[]  IOutMin=[]  IOutMax=[]  DOutMin=[]  DOutMax=[]  NOutMin=[]  NOutMax=[]  SumOutMin=[]  SumOutMax=[]  SaturationOutMin=[]  SaturationOutMax=[]  PParamMin=[]  PParamMax=[]  IParamMin=[]  IParamMax=[]  DParamMin=[]  DParamMax=[]  NParamMin=[]  NParamMax=[]  KbParamMin=[]  KbParamMax=[]  KtParamMin=[]  KtParamMax=[]  KbOutMin=[]  KbOutMax=[]  KtOutMin=[]  KtOutMax=[]  IntegratorOutMin=[]  IntegratorOutMax=[]  FilterOutMin=[]  FilterOutMax=[]  SumI1OutMin=[]  SumI1OutMax=[]  SumI2OutMin=[]  SumI2OutMax=[]  SumI3OutMin=[]  SumI3OutMax=[]  SumI4OutMin=[]  SumI4OutMax=[]  SumDOutMin=[]  SumDOutMax=[]  DifferentiatorOutMin=[]  DifferentiatorOutMax=[]  FilterDiffOutCoefMin=[]  FilterDiffOutCoefMax=[]  ReciprocalOutMin=[]  ReciprocalOutMax=[]  SumDenOutMin=[]  SumDenOutMax=[]  SumNumOutMin=[]  SumNumOutMax=[]  DivideOutMin=[]  DivideOutMax=[]  IntegratorContinuousStateAttributes=''  IntegratorStateMustResolveToSignalObject=off  IntegratorRTWStateStorageClass=Auto  FilterContinuousStateAttributes=''  FilterStateMustResolveToSignalObject=off  FilterRTWStateStorageClass=Auto  ParallelPVariant=Passthrough  IdealPVariant=InternalParameters  IVariant=InternalParameters  DVariant=InternalParameters  IntegratorVariant=Continuous  SatVariant=Disabled  AWVariant=Passthrough  PCopyVariant=Disabled  TRVariant=Disabled  FdbkBlocksVariant=Forward  IdealPFdbkVariant=Disabled  SatFdbkVariant=Disabled  DerivativeFilterVariant=ContFilter  NVariant=InternalParameters  NCopyVariant=Disabled  FilterICVariant=InternalICsFilter  IntegratorICVariant=InternalICs  ExternalResetVariant=Disabled  TRSumVariant=Passthrough  SumFdbkVariant=Disabled  SumVariant=Sum_PID
  PID Controller9 : simulink/Continuous/PID Controller  Controller=PID  Form=Ideal  TimeDomain=Continuous-time  SampleTime=-1  IntegratorMethod=Forward Euler  FilterMethod=Forward Euler  ControllerParametersSource=internal  P=-0.04  I=0.0001  D=0  UseFilter=on  N=100  TunerSelectOption=Transfer Function Based (PID Tuner App)  InitialConditionSource=internal  InitialConditionForIntegrator=-0.1  InitialConditionForFilter=0  DifferentiatorICPrevScaledInput=0  ExternalReset=none  TrackingMode=off  Kt=1  LimitOutput=off  UpperSaturationLimit=inf  LowerSaturationLimit=-inf  LinearizeAsGain=on  AntiWindupMode=none  Kb=1  POutMin=[]  POutMax=[]  IOutMin=[]  IOutMax=[]  DOutMin=[]  DOutMax=[]  NOutMin=[]  NOutMax=[]  SumOutMin=[]  SumOutMax=[]  SaturationOutMin=[]  SaturationOutMax=[]  PParamMin=[]  PParamMax=[]  IParamMin=[]  IParamMax=[]  DParamMin=[]  DParamMax=[]  NParamMin=[]  NParamMax=[]  KbParamMin=[]  KbParamMax=[]  KtParamMin=[]  KtParamMax=[]  KbOutMin=[]  KbOutMax=[]  KtOutMin=[]  KtOutMax=[]  IntegratorOutMin=[]  IntegratorOutMax=[]  FilterOutMin=[]  FilterOutMax=[]  SumI1OutMin=[]  SumI1OutMax=[]  SumI2OutMin=[]  SumI2OutMax=[]  SumI3OutMin=[]  SumI3OutMax=[]  SumI4OutMin=[]  SumI4OutMax=[]  SumDOutMin=[]  SumDOutMax=[]  DifferentiatorOutMin=[]  DifferentiatorOutMax=[]  FilterDiffOutCoefMin=[]  FilterDiffOutCoefMax=[]  ReciprocalOutMin=[]  ReciprocalOutMax=[]  SumDenOutMin=[]  SumDenOutMax=[]  SumNumOutMin=[]  SumNumOutMax=[]  DivideOutMin=[]  DivideOutMax=[]  IntegratorContinuousStateAttributes=''  IntegratorStateMustResolveToSignalObject=off  IntegratorRTWStateStorageClass=Auto  FilterContinuousStateAttributes=''  FilterStateMustResolveToSignalObject=off  FilterRTWStateStorageClass=Auto  ParallelPVariant=Passthrough  IdealPVariant=InternalParameters  IVariant=InternalParameters  DVariant=InternalParameters  IntegratorVariant=Continuous  SatVariant=Disabled  AWVariant=Passthrough  PCopyVariant=Disabled  TRVariant=Disabled  FdbkBlocksVariant=Forward  IdealPFdbkVariant=Disabled  SatFdbkVariant=Disabled  DerivativeFilterVariant=ContFilter  NVariant=InternalParameters  NCopyVariant=Disabled  FilterICVariant=InternalICsFilter  IntegratorICVariant=InternalICs  ExternalResetVariant=Disabled  TRSumVariant=Passthrough  SumFdbkVariant=Disabled  SumVariant=Sum_PID
  Product{1..27} (27 alike) : Product
  Señal de control{,1,3..4,6,8,12..15,17,19} (12 alike) : Scope
  "Señal de control    " : Scope
  Señal de control{2,5,7,9,16,18,20} (7 alike) : Scope  NumInputPorts=2
  Step : Step  Time=10  Before=7  After=4  SampleTime=0
  Sum{1..2,4..9,11..15,17..20,22..26,28..31,33..40,42..45,47..50,52..56,58..60,62..71,73..78,80..82,84..90,92..97,99..110,112..116,118..121,123..126,128..135,137,139..146,148..149,151..158,160..164} (139 alike) : Sum  Inputs=|+-
  Sum{3,10,16,21,27,32,41,46,51,57,61,72,79,83,91,98,111,117,122,127,136,138,147,150,159} (25 alike) : Sum  Inputs=|++
  Switch : Switch  Criteria=u2 > Threshold  Threshold=7
  U (ins. exógena) cte{1,3,5,7,10} (5 alike) : Constant  Value=0
  U (ins. exógena) cte{2,4,6,8,11} (5 alike) : Constant  Value=0.185
  glucosa tras ingesta{1..4,6..10,12..13,15,17..18,20,22..28} (22 alike) : Scope  NumInputPorts=2
  glucosa tras ingesta11 : Scope  NumInputPorts=4
  glucosa tras ingesta14 : Scope  NumInputPorts=5
  glucosa tras ingesta16 : Scope  NumInputPorts=4
  glucosa tras ingesta21 : Scope  NumInputPorts=4
  glucosa tras ingesta29 : Scope  NumInputPorts=3
  glucosa tras ingesta5 : Scope  NumInputPorts=5
  grafica insulina{1..14,16..23} (22 alike) : Scope  NumInputPorts=2
  grafica insulinas : Scope  NumInputPorts=5
  i(T)1 : Constant  Value=12
  i(T)6 : Constant  Value=12
  insulina activa{1..14,16..25} (24 alike) : Scope
  mODELO ORIGINAL1 : Scope  NumInputPorts=2
  mODELO ORIGINAL6 : Scope  NumInputPorts=2
  p4 = n : Gain  Gain=n
  p5 : Constant  Value=7
  p6 : Gain  Gain=p6
  "referencia glucosa " : Constant  Value=7
  referencia glucosa = Gb{,1..5,7..11} (11 alike) : Constant  Value=7
  referencia glucosa = Gb12 : Constant  Value=6
  wires:
  Gain64/1 -> Sum56/2
  Gain18/1 -> Error glucémico2/2, Error glucémico1/1  "Error regulador P"
  Sum6/1 -> Integrator1/1
  Glucosa basal11/1 -> Gain73/1, Gain72/1  "glucosa basal"
  Sum9/1 -> Sum12/1
  PID Controller/1 -> Señal de control2/1, Señal de control/1, Divide1/1  "Control regulador PI"
  Integrator28/1 -> grafica insulinas/1, grafica insulina14/1, Gain67/1, Sum55/1  "Sin insulina exógena)"
  Gain9/1 -> Error glucémico2/1, Error glucémico/1  "Error regulador PI"
  Constant4/1 -> Divide2/2
  Gain3/1 -> glucosa tras ingesta5/2, Glucosa con regulador/3, glucosa tras ingesta14/3, glucosa tras ingesta1/1  "Regulador P (prueba y error)"
  Product2/1 -> Sum12/2
  Integrator33/1 -> insulina activa11/1, Product11/2, Gain74/1  "X(t)"
  Sum59/1 -> Gain69/1
  Integrator2/1 -> Sum7/2, Gain3/1, Product1/1, Gain1/1  "G(t)"
  Gain65/1 -> Sum58/1
  Product1/1 -> Sum5/2
  Insulina basal11/1 -> grafica insulinas/5, grafica insulina12/2, Sum59/2  "Insulina basal"
  Gain73/1 -> Sum61/2
  Product11/1 -> Sum63/2
  Insulina basal1/1 -> grafica insulina1/2, Sum1/2  "Regulador P"
  Sum14/1 -> PID Controller1/1, Gain18/1  "error(ref-actual)"
  Sum57/1 -> Integrator29/1
  Constant22/1 -> Divide11/2
  Gain70/1 -> Glucosa con regulador/2, glucosa tras ingesta14/2, glucosa tras ingesta10/1  "Ingesta con insulina exógena"
  Sum12/1 -> Sum10/1
  referencia glucosa = Gb/1 -> Sum7/1  "referencia"
  Integrator32/1 -> Gain70/1, Product11/1, Gain68/1  "G(t)"
  Gain11/1 -> Sum11/1
  Sum60/1 -> Sum63/1
  Clock2/1 -> Ingesta 75 g2/1(in)
  Sum3/1 -> Integrator2/1
  Gain13/1 -> Sum13/2
  Clock11/1 -> Ingesta 75 g11/1(in)
  referencia glucosa = Gb1/1 -> Sum14/1  "referencia"
  Sum5/1 -> Sum3/1
  Integrator31/1 -> grafica insulina12/1, grafica insulinas/2, Gain71/1, Sum59/1  "Insulina exógena (cte.)"
  Gain68/1 -> Sum60/2
  Glucosa basal2/1 -> Gain15/1, Gain14/1  "glucosa basal"
  Sum10/1 -> Integrator5/1
  Divide1/1 -> Sum6/1
  U (ins. exógena) cte10/1 -> Divide10/1
  Gain15/1 -> Sum10/2
  Insulina basal2/1 -> grafica insulina2/2, Sum8/2  "insulina basal"
  Sum61/1 -> Integrator32/1
  Glucosa basal1/1 -> Gain6/1, Gain5/1  "glucosa basal"
  Gain1/1 -> Sum2/2
  Integrator4/1 -> grafica insulinas/4, grafica insulina2/1, Gain13/1, Sum8/1  "Regulador PI (Prueba y error)"
  Gain10/1 -> Sum9/2
  Sum13/1 -> Integrator4/1
  Divide2/1 -> Sum13/1
  Gain12/1 -> glucosa tras ingesta14/4, glucosa tras ingesta5/3, glucosa tras ingesta2/1  "Regulador PI (prueba y error)"
  Integrator5/1 -> Sum14/2, Gain12/1, Product2/1, Gain10/1  "G(t)"
  Ingesta 75 g2/1(D) -> Grafica ingesta D2/1, Sum9/1
  Sum4/1 -> Integrator3/1
  PID Controller1/1 -> Divide2/1, Señal de control2/2, Señal de control1/1  "Control regulador P"
  Sum11/1 -> Integrator6/1
  Gain14/1 -> glucosa tras ingesta2/2  "glucosa basal diabetico"
  Integrator1/1 -> grafica insulinas/3, grafica insulina1/1, Gain4/1, Sum1/1  "Regulador P (Prueba y Error)"
  Sum8/1 -> Gain11/1
  Sum7/1 -> PID Controller/1, Gain9/1  "error(ref-actual)"
  Integrator3/1 -> insulina activa1/1, Product1/2, Gain7/1  "X(t)"
  Gain16/1 -> Sum11/2
  Sum1/1 -> Gain2/1
  Gain5/1 -> glucosa tras ingesta1/2  "glucosa basal diabetico"
  Gain2/1 -> Sum4/1
  Integrator29/1 -> Gain66/1, Product10/1, Gain64/1  "G(t)"
  U (ins. exógena) cte11/1 -> Divide11/1
  Gain71/1 -> Sum64/2
  Sum63/1 -> Sum61/1
  Gain72/1 -> glucosa tras ingesta14/5, Glucosa con regulador/4, glucosa tras ingesta10/2  "glucosa basal"
  Sum55/1 -> Gain65/1
  Ingesta 75 g11/1(D) -> Grafica ingesta D11/1, Sum60/1
  Gain74/1 -> Sum62/2
  Clock1/1 -> Ingesta 75 g1/1(in)
  Sum56/1 -> Sum65/1
  Sum65/1 -> Sum57/1
  Sum64/1 -> Integrator31/1
  Insulina basal10/1 -> grafica insulina14/2, Sum55/2  "insulina basal"
  Sum66/1 -> Integrator28/1
  Gain67/1 -> Sum66/2
  Constant2/1 -> Divide1/2
  Gain6/1 -> Sum3/2
  Divide11/1 -> Sum64/1
  Ingesta 75 g10/1(D) -> Grafica ingesta D10/1, Sum56/1
  Glucosa basal10/1 -> Gain76/1, Gain75/1  "glucosa basal"
  Sum2/1 -> Sum5/1
  Clock10/1 -> Ingesta 75 g10/1(in)
  Divide10/1 -> Sum66/1
  Gain75/1 -> glucosa tras ingesta9/2  "glucosa basal diabetico"
  Integrator30/1 -> insulina activa10/1, Product10/2, Gain77/1  "X(t)"
  Sum62/1 -> Integrator33/1
  Gain76/1 -> Sum57/2
  Sum58/1 -> Integrator30/1
  Gain4/1 -> Sum6/2
  Ingesta 75 g1/1(D) -> Grafica ingesta D1/1, Sum2/1
  Gain77/1 -> Sum58/2
  Gain69/1 -> Sum62/1
  Constant20/1 -> Divide10/2
  Gain7/1 -> Sum4/2
  Integrator6/1 -> insulina activa2/1, Product2/2, Gain16/1  "X(t)"
  Gain66/1 -> glucosa tras ingesta9/1, Glucosa con regulador/1, glucosa tras ingesta14/1  "Ingesta"
  Product10/1 -> Sum65/2
  referencia glucosa = Gb3/1 -> Sum20/1  "referencia"
  Gain33/1 -> glucosa tras ingesta7/1  "Ingesta"
  Product4/1 -> Sum36/2
  Integrator18/1 -> insulina activa6/1, Product6/2, Gain24/1  "X(t)"
  Gain36/1 -> Sum33/1
  Gain45/1 -> Sum28/2
  Constant8/1 -> Divide4/2
  Integrator12/1 -> insulina activa4/1, Product4/2, Gain45/1  "X(t)"
  Sum28/1 -> Integrator12/1
  Gain44/1 -> Sum27/2
  Divide4/1 -> Sum37/1
  Clock4/1 -> Ingesta 75 g4/1(in)
  Gain43/1 -> glucosa tras ingesta7/2  "glucosa basal diabetico"
  Gain34/1 -> Sum37/2
  Divide5/1 -> Sum35/1
  Sum37/1 -> Integrator9/1
  Insulina basal4/1 -> grafica insulina5/2, Sum25/2  "insulina basal"
  Sum36/1 -> Sum27/1
  Sum35/1 -> Integrator13/1
  Sum26/1 -> Sum36/1
  Ingesta 75 g5/1(D) -> Grafica ingesta D5/1, Sum31/1
  Gain40/1 -> glucosa tras ingesta4/2  "glucosa basal"
  Sum33/1 -> Integrator15/1
  Gain39/1 -> Sum35/2
  U (ins. exógena) cte2/1 -> Divide5/1
  Sum34/1 -> Sum32/1
  Integrator10/1 -> Gain33/1, Product4/1, Gain31/1  "G(t)"
  Gain24/1 -> Sum17/2
  Glucosa basal4/1 -> Gain44/1, Gain43/1  "glucosa basal"
  Sum39/1 -> Gain19/1
  Gain22/1 -> glucosa tras ingesta6/2  "glucosa basal diabetico"
  PID Controller3/1 -> Divide6/1, Señal de control5/2, Señal de control4/1  "Control regulador P"
  Sum17/1 -> Integrator18/1
  Gain17/1 -> Sum40/2
  Integrator16/1 -> grafica insulina6/1, Gain21/1, Sum39/1  "I(t)"
  Divide6/1 -> Sum19/1
  Sum19/1 -> Integrator16/1
  Sum32/1 -> Integrator14/1
  U (ins. exógena) cte1/1 -> Divide4/1
  Glucosa basal6/1 -> Gain23/1, Gain22/1  "glucosa basal"
  Integrator13/1 -> grafica insulina4/1, Gain39/1, Sum29/1  "I(t)"
  Sum16/1 -> Integrator17/1
  Gain35/1 -> Sum31/2
  Clock5/1 -> Ingesta 75 g5/1(in)
  Gain21/1 -> Sum19/2
  Sum31/1 -> Sum34/1
  Gain19/1 -> Sum17/1
  Clock6/1 -> Ingesta 75 g6/1(in)
  Sum18/1 -> Sum16/1
  Gain23/1 -> Sum16/2
  Gain38/1 -> glucosa tras ingesta4/1  "Ingesta con insulina exógena"
  Integrator14/1 -> Gain38/1, Product5/1, Gain35/1  "G(t)"
  Constant10/1 -> Divide5/2
  Sum27/1 -> Integrator10/1
  Sum20/1 -> PID Controller3/1, Gain25/1  "error(ref-actual)"
  Product5/1 -> Sum34/2
  Insulina basal5/1 -> grafica insulina4/2, Sum29/2  "insulina basal"
  Integrator15/1 -> insulina activa5/1, Product5/2, Gain42/1  "X(t)"
  Sum29/1 -> Gain36/1
  Insulina basal6/1 -> grafica insulina6/2, Sum39/2  "insulina basal"
  Constant12/1 -> Divide6/2
  Integrator9/1 -> grafica insulina5/1, Gain34/1, Sum25/1  "I(t)"
  Gain25/1 -> Error glucémico5/2, Error glucémico4/1  "Error regulador P"
  Gain31/1 -> Sum26/2
  Sum25/1 -> Gain32/1
  Sum40/1 -> Sum18/1
  Glucosa basal5/1 -> Gain41/1, Gain40/1  "glucosa basal"
  Product6/1 -> Sum18/2
  Gain42/1 -> Sum33/2
  Gain32/1 -> Sum28/1
  Ingesta 75 g6/1(D) -> Grafica ingesta D6/1, Sum40/1
  Integrator17/1 -> Sum20/2, Gain20/1, Product6/1, Gain17/1  "G(t)"
  Gain41/1 -> Sum32/2
  Ingesta 75 g4/1(D) -> Grafica ingesta D4/1, Sum26/1
  Gain20/1 -> glucosa tras ingesta5/4, glucosa tras ingesta6/1  "Regulador PI sintonizado"
  referencia glucosa = Gb5/1 -> Sum76/1  "referencia"
  Gain100/1 -> Sum83/2
  Ingesta 75 g12/1(D) -> Grafica ingesta D12/1, Sum78/1
  Gain85/1 -> glucosa tras ingesta16/2, glucosa tras ingesta17/1  "Ingesta con regulador PI SINTONIZADO"
  Ingesta 75 g14/1(D) -> Grafica ingesta D14/1, Sum90/1
  Integrator40/1 -> Sum76/2, Gain85/1, Product14/1, Gain83/1  "G(t)"
  Integrator35/1 -> insulina activa12/1, Product12/2, Gain104/1  "X(t)"
  Gain102/1 -> glucosa tras ingesta18/2  "glucosa basal diabetico"
  Divide13/1 -> Sum86/1
  Gain94/1 -> Sum88/2
  Clock12/1 -> Ingesta 75 g12/1(in)
  Sum88/1 -> Integrator42/1
  Product12/1 -> Sum87/2
  Gain93/1 -> glucosa tras ingesta18/1, glucosa tras ingesta16/1  "Ingesta"
  Constant27/1 -> Divide12/2
  Gain104/1 -> Sum80/2
  Glucosa basal13/1 -> Gain100/1, Gain99/1  "glucosa basal"
  Gain92/1 -> Sum80/1
  Product14/1 -> Sum74/2
  Gain90/1 -> Error glucémico9/2, Error glucémico8/1  "Error regulador P"
  Gain91/1 -> Sum78/2
  Gain103/1 -> Sum79/2
  Sum90/1 -> Sum74/1
  Sum77/1 -> Gain92/1
  Integrator42/1 -> grafica insulina11/1, Gain94/1, Sum77/1  "I(t)"
  Insulina basal14/1 -> grafica insulina13/2, Sum89/2  "insulina basal"
  Sum81/1 -> Gain96/1
  Insulina basal13/1 -> grafica insulina10/2, Sum81/2  "insulina basal"
  Integrator38/1 -> insulina activa13/1, Product13/2, Gain101/1  "X(t)"
  Product13/1 -> Sum85/2
  Sum76/1 -> PID Controller5/1, Gain90/1  "error(ref-actual)"
  Constant23/1 -> Divide13/2
  Gain96/1 -> Sum84/1
  Sum79/1 -> Integrator34/1
  Gain84/1 -> Sum73/1
  Integrator41/1 -> insulina activa14/1, Product14/2, Gain89/1  "X(t)"
  Sum74/1 -> Sum72/1
  Gain88/1 -> Sum72/2
  Clock14/1 -> Ingesta 75 g14/1(in)
  Integrator37/1 -> Gain97/1, Product13/1, Gain95/1  "G(t)"
  Gain95/1 -> Sum82/2
  Sum72/1 -> Integrator40/1
  Clock13/1 -> Ingesta 75 g13/1(in)
  Glucosa basal14/1 -> Gain88/1, Gain87/1  "glucosa basal"
  U (ins. exógena) cte5/1 -> Divide12/1
  Integrator39/1 -> grafica insulina13/1, Gain86/1, Sum89/1  "I(t)"
  Divide14/1 -> Sum75/1
  Sum75/1 -> Integrator39/1
  Divide12/1 -> Sum88/1
  Gain83/1 -> Sum90/2
  Gain87/1 -> glucosa tras ingesta17/2  "glucosa basal diabetico"
  PID Controller5/1 -> Divide14/1, Señal de control9/2, Señal de control8/1  "Control regulador P"
  Sum73/1 -> Integrator41/1
  Sum89/1 -> Gain84/1
  Gain86/1 -> Sum75/2
  Glucosa basal12/1 -> Gain103/1, Gain102/1  "glucosa basal"
  Gain89/1 -> Sum73/2
  Gain97/1 -> glucosa tras ingesta15/1  "Ingesta con insulina exógena"
  Sum84/1 -> Integrator38/1
  Gain98/1 -> Sum86/2
  Gain101/1 -> Sum84/2
  Sum85/1 -> Sum83/1
  Sum80/1 -> Integrator35/1
  Integrator34/1 -> Gain93/1, Product12/1, Gain91/1  "G(t)"
  Constant25/1 -> Divide14/2
  U (ins. exógena) cte6/1 -> Divide13/1
  Ingesta 75 g13/1(D) -> Grafica ingesta D13/1, Sum82/1
  Gain99/1 -> glucosa tras ingesta16/4, glucosa tras ingesta15/2  "glucosa basal"
  Sum83/1 -> Integrator37/1
  Integrator36/1 -> grafica insulina10/1, Gain98/1, Sum81/1  "I(t)"
  Sum82/1 -> Sum85/1
  Sum78/1 -> Sum87/1
  Insulina basal12/1 -> grafica insulina11/2, Sum77/2  "insulina basal"
  Sum87/1 -> Sum79/1
  Sum86/1 -> Integrator36/1
  Constant30/1 -> Divide15/2
  "Glucosa basal     "/1 -> Gain110/1, Gain109/1
  Gain111/1 -> Sum92/2
  Gain108/1 -> Sum94/2
  Sum92/1 -> Integrator45/1
  Gain109/1 -> Gráfica de la glucosa/2  "glucosa basal diabetico"
  Sum94/1 -> Integrator43/1
  Divide15/1 -> Sum94/1
  Integrator43/1 -> Gráfica de la insulina/1, Sum96/1, Gain108/1  "I(t)"
  Sum91/1 -> Integrator44/1
  Integrator45/1 -> Gráfica de la insulina activa/1, Product15/2, Gain111/1  "X(t)"
  PID Controller6/1 -> "Señal de control    "/1, Divide15/1  "Control regulador P"
  Clock15/1 -> "Ingesta    "/1(in)
  Gain106/1 -> Sum92/1
  Sum95/1 -> PID Controller6/1, Gain112/1  "error"
  Sum93/1 -> Sum91/1
  Gain110/1 -> Sum91/2
  "Insulina basal     "/1 -> Sum96/2, Gráfica de la insulina/2  "Insulina basal"
  Product15/1 -> Sum93/2
  Gain112/1 -> "Error glucémico   "/1  "Error regulador"
  Integrator44/1 -> Gain107/1, Gain105/1, Product15/1, Sum95/2  "G(t)"
  Gain105/1 -> Sum97/2
  Sum97/1 -> Sum93/1
  "Ingesta    "/1(D) -> Sum97/1, Gráfica de la ingesta/1
  Gain107/1 -> glucosa tras ingesta16/3, Gráfica de la glucosa/1
  Sum96/1 -> Gain106/1
  "referencia glucosa "/1 -> Sum95/1  "referencia"
  referencia glucosa = Gb4/1 -> Sum30/1  "referencia"
  Gain55/1 -> glucosa tras ingesta13/1  "Ingesta"
  Product7/1 -> Sum67/2
  Integrator27/1 -> insulina activa9/1, Product9/2, Gain46/1  "X(t)"
  Gain58/1 -> Sum52/1
  Gain81/1 -> Sum47/2
  Gain59/1 -> Sum42/2
  Constant14/1 -> Divide7/2
  Integrator21/1 -> insulina activa7/1, Product7/2, Gain81/1  "X(t)"
  Sum47/1 -> Integrator21/1
  Gain50/1 -> Sum49/2
  Gain80/1 -> Sum46/2
  Sum38/1 -> Sum43/1
  Divide7/1 -> Sum68/1
  Clock7/1 -> Ingesta 75 g7/1(in)
  Gain79/1 -> glucosa tras ingesta13/2  "glucosa basal diabetico"
  Gain56/1 -> Sum68/2
  Divide8/1 -> Sum54/1
  Constant13/1 -> Divide3/2
  Sum68/1 -> Integrator11/1
  Insulina basal7/1 -> grafica insulina8/2, Sum44/2  "insulina basal"
  Sum67/1 -> Sum46/1
  Sum54/1 -> Integrator22/1
  Sum45/1 -> Sum67/1
  Clock3/1 -> Ingesta 75 g3/1(in)
  Ingesta 75 g3/1(D) -> Grafica ingesta D3/1, Sum38/1
  Ingesta 75 g8/1(D) -> Grafica ingesta D8/1, Sum50/1
  Gain62/1 -> glucosa tras ingesta11/4, glucosa tras ingesta8/2  "glucosa basal"
  Sum52/1 -> Integrator24/1
  Gain61/1 -> Sum54/2
  U (ins. exógena) cte4/1 -> Divide8/1
  Sum53/1 -> Sum51/1
  Integrator19/1 -> Gain55/1, Product7/1, Gain53/1  "G(t)"
  Gain46/1 -> Sum22/2
  Gain51/1 -> glucosa tras ingesta3/2  "glucosa basal diabetico"
  Integrator20/1 -> insulina activa3/1, Product3/2, Gain59/1  "X(t)"
  Gain48/1 -> Sum42/1
  Glucosa basal7/1 -> Gain80/1, Gain79/1  "glucosa basal"
  Sum70/1 -> Gain27/1
  Sum69/1 -> PID Controller2/1, Gain82/1  "error(ref-actual)"
  Integrator7/1 -> grafica insulina3/1, Gain50/1, Sum15/1  "I(t)"
  Gain30/1 -> glucosa tras ingesta12/2  "glucosa basal diabetico"
  PID Controller4/1 -> Divide9/1, Señal de control7/2, Señal de control6/1  "Control regulador P"
  Sum22/1 -> Integrator27/1
  Gain26/1 -> Sum71/2
  Integrator25/1 -> grafica insulina9/1, Gain29/1, Sum70/1  "I(t)"
  Divide9/1 -> Sum24/1
  Sum24/1 -> Integrator25/1
  Glucosa basal3/1 -> Gain52/1, Gain51/1  "glucosa basal"
  Gain8/1 -> Sum38/2
  Sum51/1 -> Integrator23/1
  Divide3/1 -> Sum49/1
  U (ins. exógena) cte3/1 -> Divide7/1
  Glucosa basal9/1 -> Gain37/1, Gain30/1  "glucosa basal"
  Integrator22/1 -> grafica insulina7/1, Gain61/1, Sum48/1  "I(t)"
  Sum21/1 -> Integrator26/1
  Gain57/1 -> Sum50/2
  Clock8/1 -> Ingesta 75 g8/1(in)
  Gain29/1 -> Sum24/2
  Sum43/1 -> Sum41/1
  Sum50/1 -> Sum53/1
  Gain27/1 -> Sum22/1
  Clock9/1 -> Ingesta 75 g9/1(in)
  Sum41/1 -> Integrator8/1
  Sum23/1 -> Sum21/1
  Gain37/1 -> Sum21/2
  Gain60/1 -> glucosa tras ingesta8/1  "Ingesta con insulina exógena"
  Integrator23/1 -> Gain60/1, Product8/1, Gain57/1  "G(t)"
  Constant16/1 -> Divide8/2
  Sum46/1 -> Integrator19/1
  Sum30/1 -> PID Controller4/1, Gain47/1  "error(ref-actual)"
  Insulina basal3/1 -> grafica insulina3/2, Sum15/2  "insulina basal"
  Product8/1 -> Sum53/2
  Product3/1 -> Sum43/2
  Insulina basal8/1 -> grafica insulina7/2, Sum48/2  "insulina basal"
  Integrator24/1 -> insulina activa8/1, Product8/2, Gain78/1  "X(t)"
  Sum48/1 -> Gain58/1
  Insulina basal9/1 -> grafica insulina9/2, Sum70/2  "insulina basal"
  Constant18/1 -> Divide9/2
  Integrator11/1 -> grafica insulina8/1, Gain56/1, Sum44/1  "I(t)"
  PID Controller2/1 -> Señal de control7/1, Señal de control3/1, Divide3/1  "Control regulador PI"
  Sum15/1 -> Gain48/1
  Gain52/1 -> Sum41/2
  Gain47/1 -> Error glucémico7/2, Error glucémico6/1  "Error regulador P"
  Gain53/1 -> Sum45/2
  Sum44/1 -> Gain54/1
  Sum71/1 -> Sum23/1
  Sum49/1 -> Integrator7/1
  Gain82/1 -> Error glucémico7/1, Error glucémico3/1  "Error regulador PI"
  Glucosa basal8/1 -> Gain63/1, Gain62/1  "glucosa basal"
  Product9/1 -> Sum23/2
  Gain78/1 -> Sum52/2
  Gain54/1 -> Sum47/1
  Sum42/1 -> Integrator20/1
  Ingesta 75 g9/1(D) -> Grafica ingesta D9/1, Sum71/1
  Integrator26/1 -> Sum30/2, Gain28/1, Product9/1, Gain26/1  "G(t)"
  Gain63/1 -> Sum51/2
  referencia glucosa = Gb2/1 -> Sum69/1  "referencia"
  Ingesta 75 g7/1(D) -> Grafica ingesta D7/1, Sum45/1
  Gain28/1 -> glucosa tras ingesta11/2, glucosa tras ingesta12/1  "Regulador P, término disminuido"
  Gain49/1 -> glucosa tras ingesta11/1, glucosa tras ingesta3/1  "Regulador P"
  Integrator8/1 -> Sum69/2, Gain49/1, Product3/1, Gain8/1  "G(t)"
  Gain115/1 -> glucosa tras ingesta11/3, glucosa tras ingesta20/1  "Regulador P, término aumentado"
  Product16/1 -> Sum100/2
  Sum104/1 -> Sum100/1
  Gain120/1 -> Error glucémico12/1  "Error regulador P"
  Insulina basal16/1 -> grafica insulina16/2, Sum103/2  "insulina basal"
  Gain118/1 -> Sum98/2
  Sum100/1 -> Sum98/1
  Clock16/1 -> Ingesta 75 g16/1(in)
  Glucosa basal16/1 -> Gain118/1, Gain117/1  "glucosa basal"
  Integrator46/1 -> grafica insulina16/1, Gain116/1, Sum103/1  "I(t)"
  Sum101/1 -> Integrator46/1
  Divide16/1 -> Sum101/1
  Sum98/1 -> Integrator47/1
  Constant32/1 -> Divide16/2
  Gain113/1 -> Sum104/2
  Gain114/1 -> Sum99/1
  Sum99/1 -> Integrator48/1
  Gain117/1 -> glucosa tras ingesta20/2  "glucosa basal diabetico"
  Gain116/1 -> Sum101/2
  Ingesta 75 g16/1(D) -> Grafica ingesta D16/1, Sum104/1
  PID Controller7/1 -> Divide16/1, Señal de control12/1  "Control regulador P"
  Gain119/1 -> Sum99/2
  referencia glucosa = Gb7/1 -> Sum102/1  "referencia"
  Sum102/1 -> PID Controller7/1, Gain120/1  "error(ref-actual)"
  Integrator48/1 -> insulina activa16/1, Product16/2, Gain119/1  "X(t)"
  Integrator47/1 -> Sum102/2, Gain115/1, Product16/1, Gain113/1  "G(t)"
  Sum103/1 -> Gain114/1
  Integrator60/1 -> Sum107/2, Gain123/1, Product17/1, Gain121/1  "G(t)"
  Integrator61/1 -> insulina activa17/1, Product17/2, Gain127/1  "X(t)"
  Gain127/1 -> Sum137/2
  referencia glucosa = Gb10/1 -> Sum107/1  "referencia"
  PID Controller10/1 -> Divide17/1, Señal de control13/1  "Control regulador P"
  Ingesta 75 g17/1(D) -> Grafica ingesta D17/1, Sum109/1
  Gain124/1 -> Sum106/2
  Sum137/1 -> Integrator61/1
  Gain125/1 -> glucosa tras ingesta24/2  "glucosa basal diabetico"
  Integrator59/1 -> grafica insulina17/1, Gain124/1, Sum108/1  "I(t)"
  Sum106/1 -> Integrator59/1
  Gain122/1 -> Sum137/1
  Constant40/1 -> Divide17/2
  Divide17/1 -> Sum106/1
  Sum136/1 -> Integrator60/1
  Sum109/1 -> Sum105/1
  Gain128/1 -> Error glucémico13/1  "Error regulador P"
  Clock17/1 -> Ingesta 75 g17/1(in)
  Insulina basal17/1 -> grafica insulina17/2, Sum108/2  "insulina basal"
  Gain126/1 -> Sum136/2
  Gain131/1 -> glucosa tras ingesta21/2, glucosa tras ingesta22/1  "Regulador PI, término I aumentado"
  Ingesta 75 g19/1(D) -> Grafica ingesta D19/1, Sum121/1
  Gain152/1 -> Sum127/2
  Integrator57/1 -> Sum115/2, Gain131/1, Product21/1, Gain129/1  "G(t)"
  Integrator63/1 -> Sum133/2, Gain138/1, Product18/1, Gain155/1  "G(t)"
  Gain138/1 -> glucosa tras ingesta21/1, glucosa tras ingesta25/1  "Regulador PI"
  Product21/1 -> Sum113/2
  Ingesta 75 g21/1(D) -> Grafica ingesta D21/1, Sum135/1
  Gain143/1 -> Sum123/1
  Glucosa basal20/1 -> Gain152/1, Gain151/1  "glucosa basal"
  Sum120/1 -> Gain143/1
  Sum125/1 -> Integrator62/1
  Gain158/1 -> Error glucémico16/1, Error glucémico14/1  "Error regulador PI"
  Sum135/1 -> Sum113/1
  Sum107/1 -> PID Controller10/1, Gain128/1  "error(ref-actual)"
  Sum110/1 -> Gain137/1
  Gain142/1 -> Sum121/2
  Gain141/1 -> Sum117/2
  PID Controller8/1 -> Señal de control16/1, Señal de control14/1, Divide18/1  "Control regulador PI"
  Gain136/1 -> Error glucémico16/2, Error glucémico15/1  "Error regulador P"
  Integrator49/1 -> grafica insulina20/1, Gain145/1, Sum120/1  "I(t)"
  Constant38/1 -> Divide21/2
  Insulina basal21/1 -> grafica insulina21/2, Sum134/2  "insulina basal"
  Sum124/1 -> Gain147/1
  Integrator55/1 -> insulina activa20/1, Product20/2, Gain153/1  "X(t)"
  Product18/1 -> Sum119/2
  Insulina basal18/1 -> grafica insulina18/2, Sum110/2  "insulina basal"
  Insulina basal20/1 -> grafica insulina19/2, Sum124/2  "insulina basal"
  Product20/1 -> Sum129/2
  Integrator54/1 -> Gain149/1, Product20/1, Gain146/1  "G(t)"
  Constant36/1 -> Divide20/2
  Glucosa basal17/1 -> Gain126/1, Gain125/1  "glucosa basal"
  Sum122/1 -> Integrator50/1
  Sum117/1 -> Integrator63/1
  Sum113/1 -> Sum111/1
  Gain149/1 -> glucosa tras ingesta26/1  "Ingesta con insulina exógena"
  Gain146/1 -> Sum126/2
  Gain130/1 -> Sum112/1
  Clock20/1 -> Ingesta 75 g20/1(in)
  Sum126/1 -> Sum129/1
  Sum119/1 -> Sum117/1
  Integrator53/1 -> grafica insulina19/1, Gain150/1, Sum124/1  "I(t)"
  Clock21/1 -> Ingesta 75 g21/1(in)
  Gain132/1 -> Sum114/2
  Sum108/1 -> Gain122/1
  Glucosa basal21/1 -> Gain134/1, Gain133/1  "glucosa basal"
  U (ins. exógena) cte7/1 -> Divide19/1
  Glucosa basal18/1 -> Gain141/1, Gain140/1  "glucosa basal"
  Gain155/1 -> Sum116/2
  Divide21/1 -> Sum114/1
  Sum127/1 -> Integrator54/1
  Sum114/1 -> Integrator56/1
  Gain123/1 -> glucosa tras ingesta21/3, glucosa tras ingesta24/1  "Regulador PI, término I disminuido"
  Gain129/1 -> Sum135/2
  Sum112/1 -> Integrator58/1
  Gain133/1 -> glucosa tras ingesta22/2  "glucosa basal diabetico"
  PID Controller9/1 -> Divide21/1, Señal de control16/2, Señal de control15/1  "Control regulador P"
  Integrator62/1 -> grafica insulina18/1, Gain139/1, Sum110/1  "I(t)"
  Sum134/1 -> Gain130/1
  Sum133/1 -> PID Controller8/1, Gain158/1  "error(ref-actual)"
  Integrator51/1 -> insulina activa18/1, Product18/2, Gain148/1  "X(t)"
  Gain135/1 -> Sum112/2
  Gain153/1 -> Sum128/2
  Product17/1 -> Sum105/2
  Sum129/1 -> Sum127/1
  Gain137/1 -> Sum118/1
  Gain121/1 -> Sum109/2
  Ingesta 75 g20/1(D) -> Grafica ingesta D20/1, Sum126/1
  Gain134/1 -> Sum111/2
  Gain140/1 -> glucosa tras ingesta25/2  "glucosa basal diabetico"
  referencia glucosa = Gb8/1 -> Sum133/1  "referencia"
  Sum130/1 -> Integrator53/1
  Ingesta 75 g18/1(D) -> Grafica ingesta D18/1, Sum116/1
  Gain150/1 -> Sum130/2
  U (ins. exógena) cte8/1 -> Divide20/1
  Sum131/1 -> Sum122/1
  Sum121/1 -> Sum131/1
  Clock18/1 -> Ingesta 75 g18/1(in)
  Insulina basal19/1 -> grafica insulina20/2, Sum120/2  "insulina basal"
  Gain154/1 -> glucosa tras ingesta23/2  "glucosa basal diabetico"
  Sum132/1 -> Integrator49/1
  Divide20/1 -> Sum130/1
  Divide19/1 -> Sum132/1
  Constant33/1 -> Divide18/2
  Gain156/1 -> Sum122/2
  Sum111/1 -> Integrator57/1
  Sum128/1 -> Integrator55/1
  Clock19/1 -> Ingesta 75 g19/1(in)
  Gain148/1 -> Sum118/2
  Integrator50/1 -> Gain144/1, Product19/1, Gain142/1  "G(t)"
  Integrator52/1 -> insulina activa19/1, Product19/2, Gain157/1  "X(t)"
  Gain139/1 -> Sum125/2
  Sum118/1 -> Integrator51/1
  Sum116/1 -> Sum119/1
  Sum123/1 -> Integrator52/1
  Integrator56/1 -> grafica insulina21/1, Gain132/1, Sum134/1  "I(t)"
  Gain151/1 -> glucosa tras ingesta21/4, glucosa tras ingesta26/2  "glucosa basal"
  Gain145/1 -> Sum132/2
  Constant34/1 -> Divide19/2
  Product19/1 -> Sum131/2
  Gain147/1 -> Sum128/1
  Divide18/1 -> Sum125/1
  Gain157/1 -> Sum123/2
  Sum105/1 -> Sum136/1
  referencia glucosa = Gb9/1 -> Sum115/1  "referencia"
  Sum115/1 -> PID Controller9/1, Gain136/1  "error(ref-actual)"
  Gain144/1 -> glucosa tras ingesta23/1  "Ingesta"
  Glucosa basal19/1 -> Gain156/1, Gain154/1  "glucosa basal"
  Integrator58/1 -> insulina activa21/1, Product21/2, Gain135/1  "X(t)"
  Gain159/1 -> Sum144/2
  Sum139/1 -> Integrator66/1
  Glucosa basal22/1 -> Gain164/1, Gain163/1  "glucosa basal"
  Gain163/1 -> glucosa tras ingesta27/2  "glucosa basal diabetico"
  Integrator65/1 -> Sum142/2, Gain161/1, Product22/1, Gain159/1  "G(t)"
  Insulina basal22/1 -> grafica insulina22/2, Sum143/2  "insulina basal"
  Sum140/1 -> Sum138/1
  Gain160/1 -> Sum139/1
  Product22/1 -> Sum140/2
  Gain165/1 -> Sum139/2
  Sum141/1 -> Integrator64/1
  Constant44/1 -> Divide22/2
  Sum144/1 -> Sum140/1
  Integrator66/1 -> insulina activa22/1, Product22/2, Gain165/1  "X(t)"
  Divide22/1 -> Sum141/1
  referencia glucosa = Gb11/1 -> Sum142/1  "referencia"
  Gain162/1 -> Sum141/2
  PID Controller11/1 -> Divide22/1, Señal de control18/2, Señal de control17/1  "Control regulador P"
  Sum138/1 -> Integrator65/1
  Ingesta 75 g22/1(D) -> Grafica ingesta D22/1, Sum144/1
  Gain166/1 -> Error glucémico18/2, Error glucémico17/1  "Error regulador P"
  Clock22/1 -> Ingesta 75 g22/1(in)
  Gain161/1 -> glucosa tras ingesta5/5, glucosa tras ingesta27/1  "Regulador PID sintonizado"
  Gain164/1 -> Sum138/2
  Sum143/1 -> Gain160/1
  Integrator64/1 -> grafica insulina22/1, Gain162/1, Sum143/1  "I(t)"
  Sum142/1 -> PID Controller11/1, Gain166/1  "error(ref-actual)"
  Clock23/1 -> Ingesta 75 g23/1(in)
  Gain170/1 -> mODELO ORIGINAL6/2  "glucosa basal"
  Gain168/1 -> Sum148/1
  i(T)6/1 -> Sum145/1
  Sum145/1 -> Gain168/1
  Sum148/1 -> Integrator68/1
  Gain172/1 -> Sum148/2
  Gain171/1 -> Sum147/2
  Sum149/1 -> Sum147/1
  Glucosa basal23/1 -> Gain171/1, Gain170/1  "glucosa basal"
  Gain169/1 -> glucosa tras ingesta5/1, mODELO ORIGINAL6/1  "Paciente no diabético"
  Product23/1 -> Sum149/2
  Gain167/1 -> Sum146/2
  Sum146/1 -> Sum149/1
  Insulina basal23/1 -> Sum145/2  "insulina basal"
  Sum147/1 -> Integrator67/1
  Integrator67/1 -> Gain169/1, Product23/1, Gain167/1  "G(t)"
  Integrator68/1 -> insulina activa23/1, Product23/2, Gain172/1  "X(t)"
  Ingesta 75 g23/1(D) -> Grafica ingesta D23/1, Sum146/1
  Integrator70/1 -> Sum154/2, Gain175/1, Product24/1, Gain173/1  "G(t)"
  Product24/1 -> Sum152/2
  Gain174/1 -> Sum151/1
  Integrator69/1 -> grafica insulina23/1, Gain176/1, Sum155/1  "I(t)"
  Sum154/1 -> PID Controller12/1, Gain180/1  "error(ref-actual)"
  Gain175/1 -> glucosa tras ingesta29/2, glucosa tras ingesta28/1  "Paciente diabético"
  Gain177/1 -> glucosa tras ingesta28/2, glucosa tras ingesta29/3  "Glucosa basal"
  Glucosa basal24/1 -> Gain178/1, Gain177/1  "glucosa basal"
  Sum155/1 -> Gain174/1
  Sum152/1 -> Sum150/1
  Sum156/1 -> Sum152/1
  Gain178/1 -> Sum150/2
  Gain173/1 -> Sum156/2
  Gain180/1 -> Error glucémico20/2, Error glucémico19/1  "Error regulador P"
  Divide23/1 -> Sum153/1
  PID Controller12/1 -> Divide23/1, Señal de control20/2, Señal de control19/1  "Control regulador P"
  Clock24/1 -> Ingesta 75 g24/1(in)
  Insulina basal24/1 -> grafica insulina23/2, Sum155/2  "insulina basal"
  Integrator71/1 -> insulina activa24/1, Product24/2, Gain179/1  "X(t)"
  Sum151/1 -> Integrator71/1
  Sum153/1 -> Integrator69/1
  Sum150/1 -> Integrator70/1
  referencia glucosa = Gb12/1 -> Sum154/1  "referencia"
  Gain176/1 -> Sum153/2
  Gain179/1 -> Sum151/2
  Constant47/1 -> Divide23/2
  Constant46/1 -> Sum156/1
  Gain185/1 -> Sum159/2
  Glucosa basal25/1 -> Gain185/1, Gain184/1  "glucosa basal"
  Sum164/1 -> Sum159/1
  Integrator72/1 -> Gain183/1, Sum160/1, Switch/2, Product25/1, Gain181/1  "G(t)"
  Product25/1 -> Sum164/2
  Sum157/1 -> Gain182/1
  Gain182/1 -> Sum163/1
  Switch/1 -> Product27/2
  p5/1 -> Sum160/2  "glucosa basal"
  Integrator73/1 -> Sum157/1, INSULINA/1, Sum161/1  "Insulina con insulina variable"
  Glucosa basal27/1 -> Switch/3  "glucosa basal"
  Gain181/1 -> Sum158/2
  p4 = n/1 -> Sum162/2
  Sum163/1 -> Integrator74/1
  Clock/1 -> Product26/1
  p6/1 -> Product26/2
  Clock25/1 -> Ingesta 75 g25/1(in)
  Glucosa basal26/1 -> Switch/1  "glucosa basal"
  Gain184/1 -> mODELO ORIGINAL1/2  "Glucosa basal"
  "Glucosa "/1 -> INSULINA/2  "Insulina Basal"
  Constant48/1 -> Grafica ingesta D25/1, Sum158/1
  Product26/1 -> Product27/1
  Ib/1 -> Sum161/2  "glucosa basal"
  Sum158/1 -> Sum164/1
  Insulina basal25/1 -> Sum157/2  "insulina basal"
  Sum159/1 -> Integrator72/1
  Product27/1 -> Sum162/1
  Sum161/1 -> p4 = n/1
  Gain183/1 -> glucosa tras ingesta29/1, mODELO ORIGINAL1/1  "Paciente no diabético"
  Integrator74/1 -> insulina activa25/1, Product25/2, Gain186/1  "Insulina activa con insulina variable"
  Gain186/1 -> Sum163/2
  Sum160/1 -> p6/1
  Sum162/1 -> Integrator73/1
